simulink model "P44"  (R2015b)
settings: Solver=VariableStepAuto  StartTime=0.0  StopTime=30  RelTol=1e-3
libraries: fl_lib x10, nesl_utility x3
settings Model: Creator=xmax1946  LastModifiedBy=xmax1946

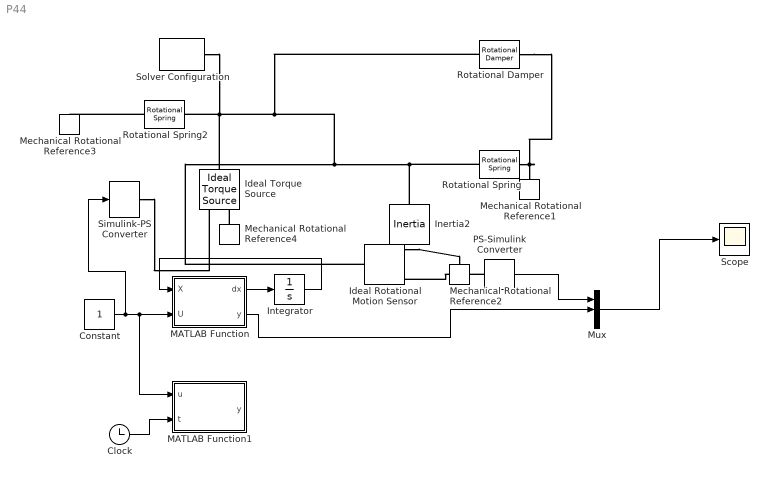
== system P44 ==
  Clock : Clock
  Constant : Constant
  Ideal Rotational Motion Sensor : fl_lib/Mechanical/Mechanical Sensors/Ideal Rotational Motion Sensor  offset=0 rad
  Ideal Torque Source : fl_lib/Mechanical/Mechanical Sources/Ideal Torque Source
  Inertia2 : fl_lib/Mechanical/Rotational Elements/Inertia  inertia=1300 kg*m^2  w_specify=off  w_priority=None  w=0 rad/s  t_specify=off  t_priority=None  t=0 N*m
  Integrator : Integrator  InitialCondition=[0;0]
  MATLAB Function : MATLAB Function  TreatAsAtomicUnit=on
  MATLAB Function1 : MATLAB Function  TreatAsAtomicUnit=on
  Mechanical Rotational Reference{1..4} (4 alike) : fl_lib/Mechanical/Rotational Elements/Mechanical Rotational Reference
  Mux : Mux  Inputs=3
  PS-Simulink Converter : nesl_utility/PS-Simulink Converter  PhysicalDomain=network_engine_domain  SubClassName=ps_output  LeftPortType=input  RightPortType=output  PseudoPeriodic=off  Frequencies=[]  Unit=1  AffineConversion=off
  Rotational Damper : fl_lib/Mechanical/Rotational Elements/Rotational Damper  D=(1000/25)*100 N*m/(rad/s)  w_specify=off  w_priority=None  w=0 rad/s  t_specify=off  t_priority=None  t=0 N*m
  Rotational Spring : fl_lib/Mechanical/Rotational Elements/Rotational Spring  spr_rate=250 N*m/rad  w_specify=off  w_priority=None  w=0 rad/s  t_specify=off  t_priority=None  t=0 N*m  phi_specify=off  phi_priority=None  phi=0 rad
  Rotational Spring2 : fl_lib/Mechanical/Rotational Elements/Rotational Spring  spr_rate=3*100 N*m/rad  w_specify=off  w_priority=None  w=0 rad/s  t_specify=off  t_priority=None  t=0 N*m  phi_specify=off  phi_priority=None  phi=0 rad
  Scope : Scope
  Simulink-PS Converter : nesl_utility/Simulink-PS Converter  PhysicalDomain=network_engine_domain  SubClassName=ps_input  LeftPortType=input  RightPortType=output  PseudoPeriodic=off  Frequencies=[]  NoiseDistribution=none  NoiseParameters=[]  Unit=1  AffineConversion=off  InputFiltering=off  SimscapeFilterOrder=1  InputFilterTimeConstant=0.001  UdotUserProvided=1
  Solver Configuration : nesl_utility/Solver Configuration  PhysicalDomain=network_engine_domain  SubClassName=solver  LeftPortType=input  RightPortType=generic  Accelerate=off  Tones=[]  Harmonics=[]  SimulateNoise=off  Profile=off  UseLocalSampling=off  EnableSwitchedLinearOptims=on  FrequencyDomain=off  UseCCode=off  RelTol=0.001  AbsTol=1e-06  MinStep=1e-09  ToWorkspace=off  RevertToSquareIcSolve=off  NumHomotopyIterations=100  PhasorMode=off  PhasorModeNumHarmonics=1  DoDC=off  ResidualTolerance=1e-09  UseLocalSolver=off  LocalSolverChoice=NE_BACKWARD_EULER_ADVANCER  LocalSolverSampleTime=0.001  DoFixedCost=off  MaxNonlinIter=3  MaxModeIter=2  LinearAlgebra=Sparse  DelaysMemoryBudget=1024  AutomaticFiltering=on  FilteringTimeConstant=0.001
  wires:
  Constant/1 -> Simulink-PS Converter/1, MATLAB Function1/1(u), MATLAB Function/2(U)
  MATLAB Function/1(dx) -> Integrator/1
  Integrator/1 -> MATLAB Function/1(X)
  PS-Simulink Converter/1 -> Mux/1
  Mux/1 -> Scope/1
  MATLAB Function/2(y) -> Mux/2
  Clock/1 -> MATLAB Function1/2(t)
  connections:
  Simulink-PS Converter/RConn1 -- Ideal Torque Source/RConn1
  Inertia2/LConn1 -- Rotational Spring/LConn1 -- Ideal Rotational Motion Sensor/LConn1 -- Rotational Damper/LConn1 -- Ideal Torque Source/LConn1 -- Solver Configuration/RConn1 -- Rotational Spring2/RConn1
  Rotational Spring2/LConn1 -- Mechanical Rotational Reference3/LConn1
  Ideal Rotational Motion Sensor/RConn1 -- Mechanical Rotational Reference2/LConn1
  PS-Simulink Converter/LConn1 -- Ideal Rotational Motion Sensor/RConn3
  Mechanical Rotational Reference4/LConn1 -- Ideal Torque Source/RConn2
  Rotational Damper/RConn1 -- Rotational Spring/RConn1 -- Mechanical Rotational Reference1/LConn1

== matlab function P44/MATLAB Function1 ==
  data: u input; y output; t input
function y = fcn(u,t)
if(t==0)
y=- 1.1034745181364905998431816682016e-35*u*exp(-1.5384615384615384615384615384615*t)*(1.7329349527450844592011026772826e33*exp(1.3941976123378352386480199154009*t) - 1.7329349527450844592011026772826e33*exp(1.5384615384615384615384615384615*t) + 85246865436733722617079140899464.0*exp(1.5384615384615384615384615384615*t) - 85246865436733722617079140899465.0*exp(-1.3941976123378352386480199154009*t)) - 0.00000038069943061538309305470069760609;
else
y=- 1.1034745181364905998431816682016e-35*u*exp(-1.5384615384615384615384615384615*t)*(1.7329349527450844592011026772826e33*exp(1.3941976123378352386480199154009*t) - 1.7329349527450844592011026772826e33*exp(1.5384615384615384615384615384615*t) + 85246865436733722617079140899464.0*exp(1.5384615384615384615384615384615*t) - 85246865436733722617079140899465.0*exp(-1.3941976123378352386480199154009*t)) - 0.00000038069943061538309305470069760609;
end

== matlab function P44/MATLAB Function ==
  data: dx output; X input; y output; U input
function [dx,y] = fss(X,U)
A=[0,1;-550/1300,-4000/1300];
B=[0;10/1300];
C=[1/10,0];
u=U;
dx=A*X+B*u;
y=C*X;
% 
% t=1
% (2^(1/2)*73^(1/2)*sinh((3*2^(1/2)*73^(1/2)*t)/26)*exp(-(20*t)/13))/2190
